simulink model "Nonlinear_GSSA"  (R2016a)
settings: Solver=VariableStepAuto  StartTime=0.0  StopTime=10  RelTol=1e-3
values from neighbouring files (symbols this model uses):
  ba = 3e-4    (= 0.0003)    [Ini_non_lin.m]    (also in System_Identification.m = 0.1; The_whole_system_conected.m)
  bl = 0.001    [Ini_non_lin.m]    (also in System_Identification.m = 0.1; The_whole_system_conected.m)
  Jm = 1.1472    [Identification.m]    (also in Ini_non_lin.m = 0.0006375; System_Identification.m = 0.0006375; The_whole_system_conected.m = 0.0006375)
  kb = 4.875    [Ini_non_lin.m]    (also in System_Identification.m; The_whole_system_conected.m)
  Ke = 1.131    [Identification.m]    (also in Ini_non_lin.m = 0.0169; System_Identification.m = 1.13; The_whole_system_conected.m = 0.0169)
  ks = 48.75    [Ini_non_lin.m]    (also in System_Identification.m; The_whole_system_conected.m)
  Kt = 1.395    [Identification.m]    (also in Ini_non_lin.m = 191.3; System_Identification.m = 1.39; The_whole_system_conected.m = 191.3)
  l = 80    [Ini_non_lin.m]    (also in System_Identification.m; The_whole_system_conected.m)
  Ld = 3.427e-3    (= 0.003427)    [Identification.m]    (also in Ini_non_lin.m; System_Identification.m; The_whole_system_conected.m)
  Lq = 3.334e-3    (= 0.003334)    [Identification.m]    (also in Ini_non_lin.m; System_Identification.m; The_whole_system_conected.m)
  M = 10    [Ini_non_lin.m]    (also in System_Identification.m; The_whole_system_conected.m)
  p = 12    [Identification.m]    (also in Ini_non_lin.m = 6; System_Identification.m = 6; The_whole_system_conected.m = 6)
  q = 9    [Ini_non_lin.m]    (also in System_Identification.m; The_whole_system_conected.m)
  r = 22.5    [Ini_non_lin.m]    (also in System_Identification.m; The_whole_system_conected.m)
  R = 0.378    [Identification.m]    (also in Ini_non_lin.m; System_Identification.m; The_whole_system_conected.m)
settings Model: Creator=Loki  LastModifiedBy=Loki

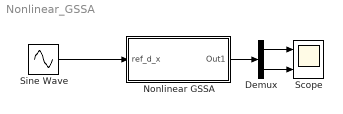
== system Nonlinear_GSSA ==
  Demux : Demux  Outputs=2
  Nonlinear GSSA : Subsystem
  Scope : Scope  NumInputPorts=2
  Sine Wave : Sin  Amplitude=8  Frequency=157  SampleTime=0
  wires:
  Nonlinear GSSA/1(Out1) -> Demux/1
  Demux/1 -> Scope/1
  Demux/2 -> Scope/2
  Sine Wave/1 -> Nonlinear GSSA/1(ref_d_x)

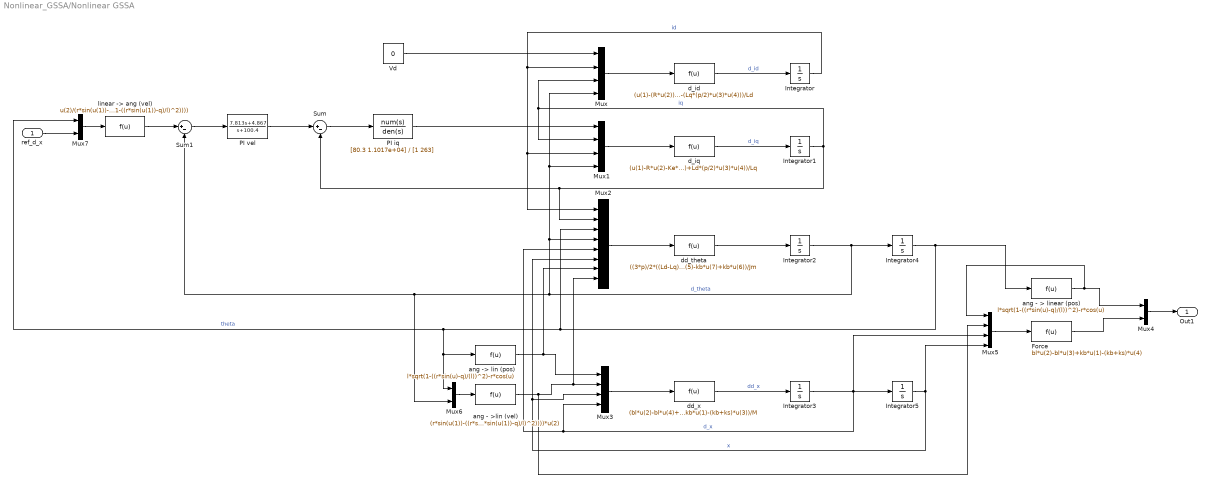
== system Nonlinear_GSSA/Nonlinear GSSA ==
  ref_d_x : Inport
  Force : Fcn  Expr=bl*u(2)-bl*u(3)+kb*u(1)-(kb+ks)*u(4)
  Integrator{,1..5} (6 alike) : Integrator
  Mux{,1,3,5} (4 alike) : Mux
  Mux2 : Mux  Inputs=8
  Mux4 : Mux  Inputs=2
  Mux6 : Mux  Inputs=2
  Mux7 : Mux  Inputs=2
  PI iq : TransferFcn  Numerator=[80.3 1.1017e+04]  Denominator=[1 263]
  PI vel : TransferFcn  Numerator=[7.813 4.867]  Denominator=[1 100.4]
  Sum : Sum  Inputs=|+-
  Sum1 : Sum  Inputs=|+-
  Vd : Constant  Value=0
  ang - > linear (pos) : Fcn  Expr=l*sqrt(1-((r*sin(u)-q)/(l))^2)-r*cos(u)
  ang - >lin (vel) : Fcn  Expr=(r*sin(u(1))-((r*sin(u(1))*cos(u(1))-r*q*cos(u(1)))/(l*sqrt(1-((r*sin(u(1))-q)/l)^2))))*u(2)
  "ang -> lin (pos)" : Fcn  Expr=l*sqrt(1-((r*sin(u)-q)/(l))^2)-r*cos(u)
  d_id : Fcn  Expr=(u(1)-(R*u(2))-(Lq*(p/2)*u(3)*u(4)))/Ld
  d_iq : Fcn  Expr=(u(1)-R*u(2)-Ke*u(4)+Ld*(p/2)*u(3)*u(4))/Lq
  dd_theta : Fcn  Expr=((3*p)/2*((Ld-Lq)*u(1)*u(2))+Kt*u(2)-ba*u(4)-(ba+bl)*u(8)+bl*u(5)-kb*u(7)+kb*u(6))/Jm
  dd_x : Fcn  Expr=(bl*u(2)-bl*u(4)+kb*u(1)-(kb+ks)*u(3))/M
  "linear -> ang (vel)" : Fcn  Expr=u(2)/(r*sin(u(1))-((r*sin(u(1))*cos(u(1))-r*q*cos(u(1)))/(l*sqrt(1-((r*sin(u(1))-q)/l)^2))))
  Out1 : Outport
  wires:
  Integrator2/1 -> Mux1/4, Mux/4, Mux2/4, Mux6/2, Sum1/2, Integrator4/1  "d_theta"
  Mux4/1 -> Out1/1
  PI iq/1 -> Mux1/1
  Vd/1 -> Mux/1
  d_id/1 -> Integrator/1  "d_id"
  Mux1/1 -> d_iq/1
  d_iq/1 -> Integrator1/1  "d_iq"
  dd_theta/1 -> Integrator2/1
  Mux2/1 -> dd_theta/1
  Mux3/1 -> dd_x/1
  dd_x/1 -> Integrator3/1  "dd_x"
  Mux/1 -> d_id/1
  Sum/1 -> PI iq/1
  PI vel/1 -> Sum/1
  "linear -> ang (vel)"/1 -> Sum1/1
  Sum1/1 -> PI vel/1
  Integrator1/1 -> Mux2/2, Sum/2, Mux/3, Mux1/2  "iq"
  ang - > linear (pos)/1 -> Mux5/1, Mux4/1
  Force/1 -> Mux4/2
  Integrator/1 -> Mux/2, Mux2/1, Mux1/3  "id"
  Integrator5/1 -> Mux3/3, Mux2/6, Mux5/4  "x"
  Integrator3/1 -> Mux3/4, Mux2/5, Integrator5/1, Mux5/3  "d_x"
  Integrator4/1 -> Mux7/1, "ang -> lin (pos)"/1, Mux6/1, Mux2/3, ang - > linear (pos)/1  "theta"
  Mux5/1 -> Force/1
  ang - >lin (vel)/1 -> Mux5/2, Mux2/8, Mux3/2
  Mux6/1 -> ang - >lin (vel)/1
  "ang -> lin (pos)"/1 -> Mux2/7, Mux3/1
  Mux7/1 -> "linear -> ang (vel)"/1
  ref_d_x/1 -> Mux7/2
